simulink model "apertura_chiusura_automatica"  (R2023b)
settings: Solver=VariableStepAuto  StartTime=0.0  StopTime=60  RelTol=1e-3
settings Model: Creator=Asus  LastModifiedBy=Asus
settings OptimizationCC: ReuseModelBlockBuffer=off

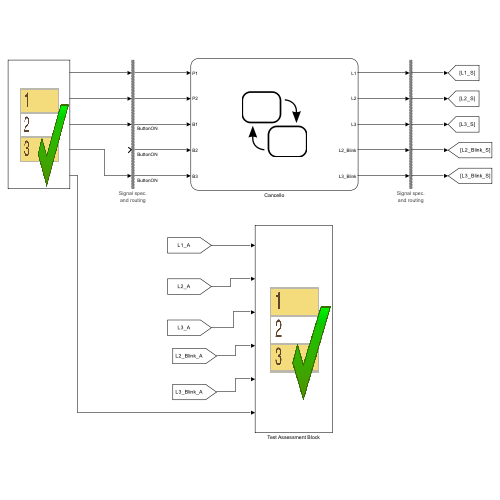
[thumbnail: Simulink's stored preview of the top-level diagram]
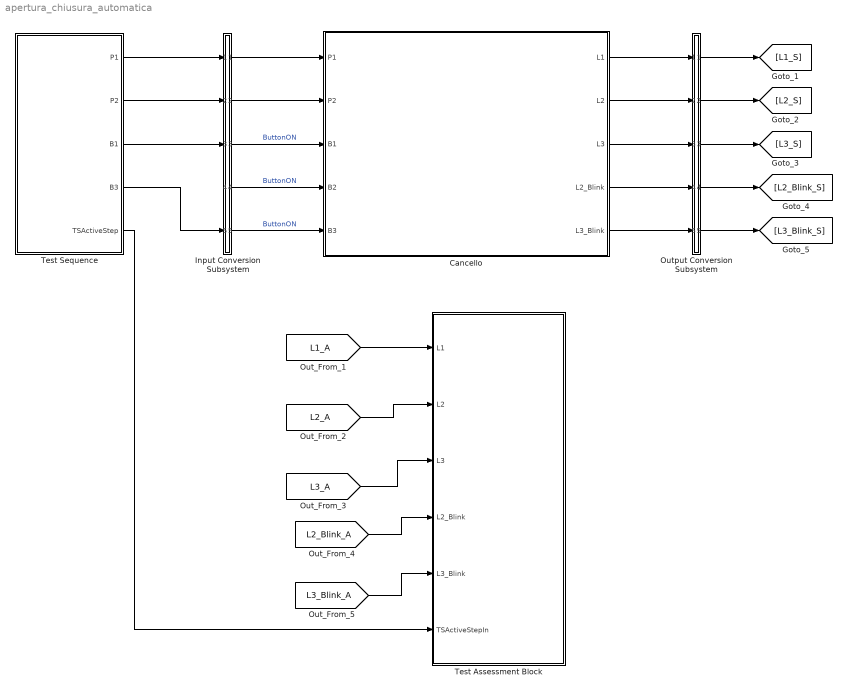
== system apertura_chiusura_automatica ==
  Cancello : Stateflow chart  TreatAsAtomicUnit=on
  Input Conversion Subsystem : Subsystem  Tag=__SLT_ICS__  Description=|
      | Signal spec.
      | and routing
      settings: AttributesFormatString=%<Description>
  Output Conversion Subsystem : Subsystem  Tag=__SLT_OCS__  Description=|
      | Signal spec.
      | and routing
      settings: AttributesFormatString=%<Description>
  Test Assessment Block : Test Sequence  Tag=__SLT_ASMT__  TreatAsAtomicUnit=on
  Test Sequence : Test Sequence  TreatAsAtomicUnit=on
  wires:
  [L1_A] -> Test Assessment Block/1(L1)
  [L2_A] -> Test Assessment Block/2(L2)
  [L3_A] -> Test Assessment Block/3(L3)
  [L2_Blink_A] -> Test Assessment Block/4(L2_Blink)
  [L3_Blink_A] -> Test Assessment Block/5(L3_Blink)
  Test Sequence/1(P1) -> Input Conversion Subsystem/1(Inport_1)
  Test Sequence/2(P2) -> Input Conversion Subsystem/2(Inport_2)
  Test Sequence/3(B1) -> Input Conversion Subsystem/3(Inport_3)
  Output Conversion Subsystem/1(Outport_1) -> [L1_S]
  Output Conversion Subsystem/2(Outport_2) -> [L2_S]
  Output Conversion Subsystem/3(Outport_3) -> [L3_S]
  Output Conversion Subsystem/4(Outport_4) -> [L2_Blink_S]
  Output Conversion Subsystem/5(Outport_5) -> [L3_Blink_S]
  Input Conversion Subsystem/1(Outport_1) -> Cancello/1(P1)
  Input Conversion Subsystem/2(Outport_2) -> Cancello/2(P2)
  Input Conversion Subsystem/3(Outport_3) -> Cancello/3(B1)  "ButtonON"
  Input Conversion Subsystem/4(Outport_4) -> Cancello/4(B2)  "ButtonON"
  Input Conversion Subsystem/5(Outport_5) -> Cancello/5(B3)  "ButtonON"
  Cancello/1(L1) -> Output Conversion Subsystem/1(Inport_1)
  Cancello/2(L2) -> Output Conversion Subsystem/2(Inport_2)
  Cancello/3(L3) -> Output Conversion Subsystem/3(Inport_3)
  Cancello/4(L2_Blink) -> Output Conversion Subsystem/4(Inport_4)
  Cancello/5(L3_Blink) -> Output Conversion Subsystem/5(Inport_5)
  Test Sequence/5(TSActiveStep) -> Test Assessment Block/6(TSActiveStepIn)
  Test Sequence/4(B3) -> Input Conversion Subsystem/5(Inport_5)

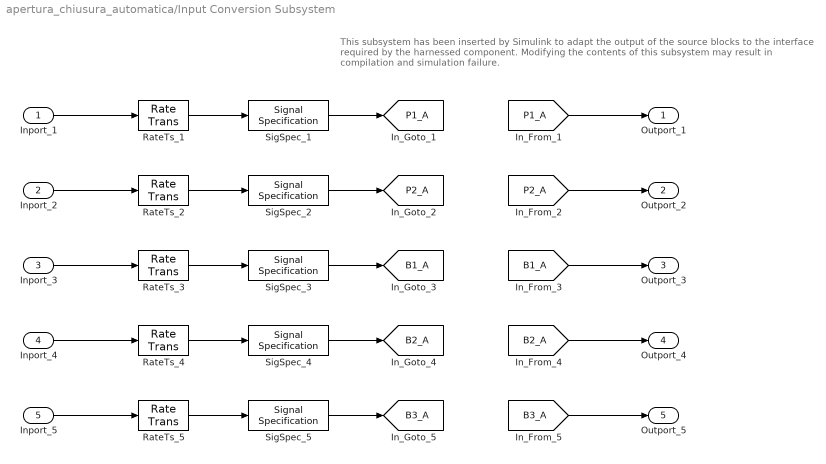
== system apertura_chiusura_automatica/Input Conversion Subsystem ==
  note: This subsystem has been inserted by Simulink to adapt the output of the source blocks to the interface required by the harnessed component.
      |  Modifying the contents of this subsystem may result in compilation and simulation failure.
  Inport_1 : Inport
  Inport_2 : Inport  Port=2
  Inport_3 : Inport  Port=3
  Inport_4 : Inport  Port=4
  Inport_5 : Inport  Port=5
  RateTs_{1..5} (5 alike) : RateTransition  OutPortSampleTime=[0, 1]
  SigSpec_{1..5} (5 alike) : SignalSpecification  OutDataTypeStr=boolean  Dimensions=[1]  SampleTime=[0, 1]
  Outport_1 : Outport
  Outport_2 : Outport  Port=2
  Outport_3 : Outport  Port=3
  Outport_4 : Outport  Port=4
  Outport_5 : Outport  Port=5
  tag scope: B1_A=global, B2_A=global, B3_A=global, P1_A=global, P2_A=global
  wires:
  [P1_A] -> Outport_1/1
  SigSpec_1/1 -> [P1_A]
  RateTs_1/1 -> SigSpec_1/1
  Inport_1/1 -> RateTs_1/1
  [P2_A] -> Outport_2/1
  SigSpec_2/1 -> [P2_A]
  RateTs_2/1 -> SigSpec_2/1
  Inport_2/1 -> RateTs_2/1
  [B1_A] -> Outport_3/1
  SigSpec_3/1 -> [B1_A]
  RateTs_3/1 -> SigSpec_3/1
  Inport_3/1 -> RateTs_3/1
  [B2_A] -> Outport_4/1
  SigSpec_4/1 -> [B2_A]
  RateTs_4/1 -> SigSpec_4/1
  Inport_4/1 -> RateTs_4/1
  [B3_A] -> Outport_5/1
  SigSpec_5/1 -> [B3_A]
  RateTs_5/1 -> SigSpec_5/1
  Inport_5/1 -> RateTs_5/1

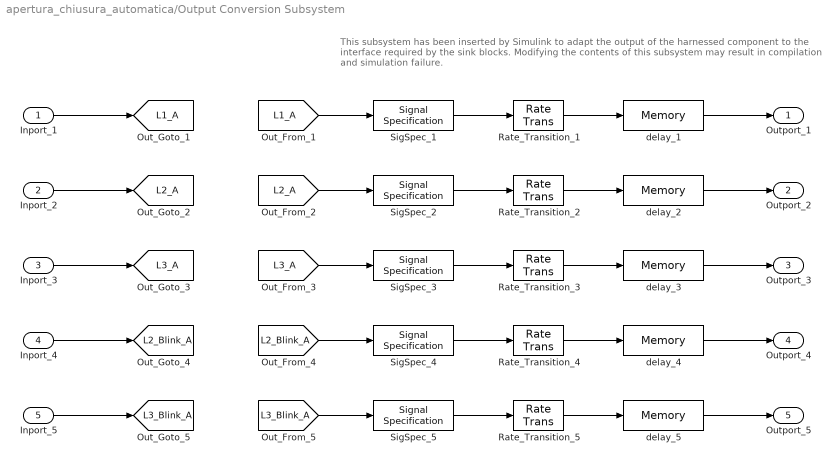
== system apertura_chiusura_automatica/Output Conversion Subsystem ==
  note: This subsystem has been inserted by Simulink to adapt the output of the harnessed component to the interface required by the sink blocks.
      |  Modifying the contents of this subsystem may result in compilation and simulation failure.
  Inport_1 : Inport
  Inport_2 : Inport  Port=2
  Inport_3 : Inport  Port=3
  Inport_4 : Inport  Port=4
  Inport_5 : Inport  Port=5
  Rate_Transition_{1..5} (5 alike) : RateTransition  OutPortSampleTimeOpt=Inherit
  SigSpec_{1..5} (5 alike) : SignalSpecification  OutDataTypeStr=boolean  Dimensions=[1]
  delay_{1..5} (5 alike) : Memory
  Outport_1 : Outport
  Outport_2 : Outport  Port=2
  Outport_3 : Outport  Port=3
  Outport_4 : Outport  Port=4
  Outport_5 : Outport  Port=5
  tag scope: L1_A=global, L2_A=global, L2_Blink_A=global, L3_A=global, L3_Blink_A=global
  wires:
  Inport_1/1 -> [L1_A]
  [L1_A] -> SigSpec_1/1
  SigSpec_1/1 -> Rate_Transition_1/1
  Rate_Transition_1/1 -> delay_1/1
  delay_1/1 -> Outport_1/1
  Inport_2/1 -> [L2_A]
  [L2_A] -> SigSpec_2/1
  SigSpec_2/1 -> Rate_Transition_2/1
  Rate_Transition_2/1 -> delay_2/1
  delay_2/1 -> Outport_2/1
  Inport_3/1 -> [L3_A]
  [L3_A] -> SigSpec_3/1
  SigSpec_3/1 -> Rate_Transition_3/1
  Rate_Transition_3/1 -> delay_3/1
  delay_3/1 -> Outport_3/1
  Inport_4/1 -> [L2_Blink_A]
  [L2_Blink_A] -> SigSpec_4/1
  SigSpec_4/1 -> Rate_Transition_4/1
  Rate_Transition_4/1 -> delay_4/1
  delay_4/1 -> Outport_4/1
  Inport_5/1 -> [L3_Blink_A]
  [L3_Blink_A] -> SigSpec_5/1
  SigSpec_5/1 -> Rate_Transition_5/1
  Rate_Transition_5/1 -> delay_5/1
  delay_5/1 -> Outport_5/1

== stateflow chart apertura_chiusura_automatica/Test Assessment Block ==
  state Run
    state VerifyInit
      verify(~L1 & ~L2 & ~L3 & ~L2_Blink & ~L3_Blink)
    state VerifyIAumentoTimerChiusura
      verify(~L1 & ~L2 & ~L3 & ~L2_Blink & ~L3_Blink)
    state VerifyRichiestaApertura
      verify(~L1 & ~L2 & ~L3 & L2_Blink & ~L3_Blink)
    state VerifyApertura
      verify(~L1 & ~L2 & ~L3 & L2_Blink & ~L3_Blink)
    state VerifyCancelloAperto
      verify(L1 & L2 & L3 & ~L2_Blink & ~L3_Blink)
    state VerifyAvvioTimer
      verify(L1 & L2 & L3 & ~L2_Blink & ~L3_Blink)
    state VerifyAvvioChiusura
      verify(~L1 && ~L2 && ~L3 && L2_Blink && ~L3_Blink)
    state VerifyChiusura
      verify(~L1 && ~L2 && ~L3 && L2_Blink && ~L3_Blink)
    state VerifyCancelloChiuso
      verify(~L1 && ~L2 && ~L3 && ~L2_Blink && ~L3_Blink)
    state Run_1
    (default) -> (junction 22)
    Run -> (junction 22)
    (junction 22) -> (junction 23) [order 1] : [TSActiveStepIn==TSActiveStepEnumH1.Init
        | ]
    (junction 23) -> VerifyInit [order 1] : [~in(Run.VerifyInit)]
    (junction 225) -> (junction 116) [order 2]
    (junction 23) -> (junction 26) [order 2]
    (junction 225) -> (junction 226) [order 1] : [TSActiveStepIn==TSActiveStepEnumH1.AumentoTimerChiusura
        | ]
    (junction 226) -> VerifyIAumentoTimerChiusura [order 1] : [~in(Run.VerifyIAumentoTimerChiusura)]
    (junction 116) -> (junction 117) [order 1] : [TSActiveStepIn==TSActiveStepEnumH1.RichiestaApertura
        | ]
    (junction 117) -> VerifyRichiestaApertura [order 1] : [~in(Run.VerifyRichiestaApertura)]
    (junction 116) -> (junction 146) [order 2]
    (junction 117) -> (junction 120) [order 2]
    (junction 146) -> (junction 147) [order 1] : [TSActiveStepIn==TSActiveStepEnumH1.Apertura
        | ]
    (junction 147) -> VerifyApertura [order 1] : [~in(Run.VerifyApertura)]
    (junction 146) -> (junction 61) [order 2]
    (junction 147) -> (junction 150) [order 2]
    (junction 61) -> (junction 62) [order 1] : [TSActiveStepIn==TSActiveStepEnumH1.CancelloAperto
        | ]
    (junction 62) -> VerifyCancelloAperto [order 1] : [~in(Run.VerifyCancelloAperto)]
    (junction 61) -> (junction 216) [order 2]
    (junction 62) -> (junction 65) [order 2]
    (junction 216) -> (junction 217) [order 1] : [TSActiveStepIn==TSActiveStepEnumH1.AvvioTimer
        | ]
    (junction 217) -> VerifyAvvioTimer [order 1] : [~in(Run.VerifyAvvioTimer)]
    (junction 216) -> (junction 207) [order 2]
    (junction 217) -> (junction 220) [order 2]
    (junction 207) -> (junction 208) [order 1] : [TSActiveStepIn==TSActiveStepEnumH1.AvvioChiusura
        | ]
    (junction 208) -> VerifyAvvioChiusura [order 1] : [~in(Run.VerifyAvvioChiusura)]
    (junction 207) -> (junction 197) [order 2]
    (junction 208) -> (junction 211) [order 2]
    (junction 197) -> (junction 198) [order 1] : [TSActiveStepIn==TSActiveStepEnumH1.Chiusura
        | ]
    (junction 198) -> VerifyChiusura [order 1] : [~in(Run.VerifyChiusura)]
    (junction 197) -> (junction 69) [order 2]
    (junction 198) -> (junction 201) [order 2]
    (junction 69) -> (junction 70) [order 1] : [TSActiveStepIn==TSActiveStepEnumH1.CancelloChiuso
        | ]
    (junction 70) -> VerifyCancelloChiuso [order 1] : [~in(Run.VerifyCancelloChiuso)]
    (junction 69) -> (junction 78) [order 2]
    (junction 70) -> (junction 73) [order 2]
    (junction 78) -> (junction 79)
    (junction 79) -> Run_1 [order 1] : [~in(Run.Run_1)]
    (junction 79) -> (junction 82) [order 2]
    (junction 226) -> (junction 229) [order 2]
    (junction 22) -> (junction 225) [order 2]
  (default) -> Run
  data: L1 input boolean size=[1]; L2 input boolean size=[1]; L3 input boolean size=[1]; L2_Blink input boolean size=[1]; L3_Blink input boolean size=[1]; TSActiveStepIn input

== stateflow chart apertura_chiusura_automatica/Test Sequence ==
  settings: sampleTime=2.4
  state Init
    %% Initialize data outputs.
    P2 = true;
    P1 = false;
    settings: description=Allo step Init il cancello si trova nello Stato di Check dove abbiamo il cancello chiuso e tutti i led spenti.
  state AumentoTimerChiusura
    B3=true;
    settings: description=|
        | A cancello chiuso viene incrementato di dieci secondi il tempo di attesa per la chiusura automatica.
        |  -> in cancello Aperto after(20,sec)
        | non viene testato l'incremento completo da 10 a 120, fino a tornare a 10 secondi
        | in quanto uguale al test apertura_chiusura_automatica
  state RichiestaApertura
    P2 = true;
    B1 = true;
    B3=false;
    settings: description=Con la pressione e il rilascio di B1 richiediamo l'apertura del cancello. il led giallo si attiva
  state Apertura
    B1 =false;
    P2 =false;
    settings: description=|
        | Step che indica il movimento del cancello. il led giallo lampeggia.
        | Questo step ha una durata di  10 secondi (tempo di apertura del cancello di default)
  state CancelloAperto
    B1 =false;
    P2 =false;
    settings: description=Non viene richiesta la di chiusura del cancello tramite B1, quindi il cancello si richiuderà dopo 20 secondi
  state AvvioTimer
    P2 =false;
    settings: description=Avvio del Timer
  state AvvioChiusura
    P2 =false;
    settings: description=Timer scaduto e inizio chiusura automatica
  state Chiusura
    B1 = false;
    settings: description=|
        | Step che indica il movimento del cancello. il led giallo lampeggia.
        | Questo step ha una durata di  10 secondi (tempo di apertura del cancello di default).
        | Nel test apertura_chiusura.automatica verrà illustrata la chiusura automatica
  state CancelloChiuso
    P2 = true;
    B1 = false;
    settings: description=Abbiamo il cancello chiuso e tutti i led spenti
  (default) -> Init
  Init -> AumentoTimerChiusura : [
      | true
      | ]
  AumentoTimerChiusura -> RichiestaApertura : [
      | true
      | ]
  RichiestaApertura -> Apertura : [
      | true
      | ]
  Apertura -> CancelloAperto : [
      | after(10,sec)
      | ]
  CancelloAperto -> AvvioTimer : [
      | after(20,sec)
      | ]
  AvvioTimer -> AvvioChiusura : [
      | true
      | ]
  AvvioChiusura -> Chiusura : [
      | true
      | ]
  Chiusura -> CancelloChiuso : [
      | after(10,sec)
      | ]
  data: P1 output boolean size=[1]; P2 output boolean size=[1]; B1 output boolean size=[1]; B3 output; TSActiveStep output Enum: TSActiveStepEnumH1

== stateflow chart apertura_chiusura_automatica/Cancello ==
  settings: executeAtInitialization=1
  state Cancello [parallel]
    settings: executionOrder=1
    state Check
      en: L1=OFF; L2=OFF; L3=OFF;L2_Blink=OFF;L3_Blink=OFF
    state Error
      state Wait1
      state ERR
        en: L1=ON
        ex: L1=OFF
      (default) -> Wait1
      Wait1 -> ERR : [after(10,sec)]
    state Close
      state Closing
        en:L2_Blink=ON; Start_T_L_C=ON;
        ex:Start_T_L_C=OFF; L2_Blink=OFF;
      state Closed
      (default) -> Closing
      Closing -> Closed : [T_L==ON && P2 == true]
    state Open
      state Opening
        en: Start_T_L_O=ON;L2_Blink=ON;
        ex:L2_Blink=OFF,Start_T_L_O=OFF
      state Opened
        en:L1=ON; L2=ON; L3=ON; Start_T_C=ON;
        du: Reset();
        ex: L1=OFF; L2=OFF; L3=OFF; Start_T_C=OFF;
      (default) -> Opening
      Opening -> Opened : [T_L == ON]
    (default) -> Check
    Check -> Open [order 2] : [B1 == ON && P1 == false || P1 == true && P2 == false]
    Close -> Error [order 2] : [T_L==ON&&P2==false]
    Check -> Close [order 1] : [P1 == false && P2 == false]
    Close -> Open [order 1] : [B1 == ON && P1 == false || in(Close.Closing) && P1==true]
    Error -> Closed : [P2==true]
    Open -> Close : [(B1 == ON || T_C == true) && P1==false]
  state Timer_T_L_O [parallel]
    settings: executionOrder=7
    state Counting
      state Count1
      state End
        en: T_L = ON
      (default) -> Timer_T_L_O.Counting.Count1
      Timer_T_L_O.Counting.Count1 -> Timer_T_L_O.Counting.End [order 1] : [after(Time_T_L,sec)]
      Timer_T_L_O.Counting.Count1 -> Timer_T_L_O.Counting.Count1 [order 2] : [RESET == ON]
    state off
      en: T_L =OFF
    (default) -> Timer_T_L_O.off
    Timer_T_L_O.off -> Timer_T_L_O.Counting : [Start_T_L_O == ON]
    Timer_T_L_O.Counting -> Timer_T_L_O.off : [Start_T_L_O == OFF]
  state Timer_T_L_C [parallel]
    settings: executionOrder=4
    state Counting
      state Count1
      state End
        en: T_L = ON
      (default) -> Timer_T_L_C.Counting.Count1
      Timer_T_L_C.Counting.Count1 -> Timer_T_L_C.Counting.End [order 1] : [after(Time_T_L,sec)]
      Timer_T_L_C.Counting.Count1 -> Timer_T_L_C.Counting.Count1 [order 2] : [RESET == ON]
    state off
      en: T_L =OFF
    (default) -> Timer_T_L_C.off
    Timer_T_L_C.off -> Timer_T_L_C.Counting : [Start_T_L_C == ON]
    Timer_T_L_C.Counting -> Timer_T_L_C.off : [Start_T_L_C == OFF]
  state Reset [function]
    (default) -> (junction 65)
    (junction 65) -> (junction 68) [order 1] : [P1==true]
    (junction 68) -> (junction 73) : {RESET=true;}
    (junction 65) -> (junction 71) [order 2] : [P1==false]
    (junction 71) -> (junction 73) : {RESET=false;}
  state Update_Time_T_L [function]
    (default) -> (junction 97)
    (junction 97) -> (junction 99) [order 1] : [Time_T_L < 120]
    (junction 99) -> (junction 107) : {Time_T_L=Time_T_L+10}
    (junction 97) -> (junction 103) [order 2] : [Time_T_L >= 120]
    (junction 103) -> (junction 107) : {Time_T_L = 10}
  state Timet_T_C [parallel]
    settings: executionOrder=5
    state Counting
      state Count1
      state End
        en: T_C = ON
      (default) -> Timet_T_C.Counting.Count1
      Timet_T_C.Counting.Count1 -> Timet_T_C.Counting.End [order 1] : [after(Time_T_C,sec)]
      Timet_T_C.Counting.Count1 -> Timet_T_C.Counting.Count1 [order 2] : [RESET == ON]
    state off
      en: T_C =OFF
    (default) -> Timet_T_C.off
    Timet_T_C.off -> Timet_T_C.Counting : [Start_T_C == ON]
    Timet_T_C.Counting -> Timet_T_C.off : [Start_T_C == OFF]
  state Update_Time_T_C [function]
    (default) -> (junction 114)
    (junction 114) -> (junction 116) [order 1] : [Time_T_C < 120]
    (junction 116) -> (junction 120) : {Time_T_C=Time_T_C + 10}
    (junction 114) -> (junction 118) [order 2] : [Time_T_C >= 120]
    (junction 118) -> (junction 120) : {Time_T_C = 10}
  state Obstacle [parallel]
    settings: executionOrder=2
    state Wait
    state OBS
      en: L3_Blink=ON;Start_T_LV=ON
      du: Reset_LV()
      ex:L3_Blink=OFF;Start_T_LV=OFF
    (default) -> Wait
    Wait -> OBS : [(in(Cancello.Close.Closed) || in(Cancello.Open.Opened) || in(Cancello.Check)) && B1==ON &&P1==true]
    OBS -> Wait : [P1==false || T_LV==ON ]
  state Update [parallel]
    settings: executionOrder=3
    state Update_TC [parallel]
      settings: executionOrder=1
      state Update_T_C
      state UP_TC
        en: Update_Time_T_C()
      (default) -> Update_T_C
      UP_TC -> Update_T_C
      Update_T_C -> UP_TC : [(in(Cancello.Close.Closed)||in(Cancello.Check)) && B3 == ON]
    state Update_TL [parallel]
      settings: executionOrder=2
      state Update_T_L
      state UP_TL
        en: Update_Time_T_L()
      (default) -> Update_T_L
      UP_TL -> Update_T_L
      Update_T_L -> UP_TL : [(in(Cancello.Close.Closed) || in(Cancello.Check)) && B2==ON]
  state Timer_LV [parallel]
    settings: executionOrder=6
    state Counting
      state Count1
      state End
        en: T_LV = ON
      (default) -> Timer_LV.Counting.Count1
      Timer_LV.Counting.Count1 -> Timer_LV.Counting.End [order 1] : [after(30,sec)]
      Timer_LV.Counting.Count1 -> Timer_LV.Counting.Count1 [order 2] : [RESET_LV==true]
    state off
      en: T_LV =OFF
    (default) -> Timer_LV.off
    Timer_LV.off -> Timer_LV.Counting : [Start_T_LV == ON]
    Timer_LV.Counting -> Timer_LV.off : [Start_T_LV == OFF]
  state Reset_LV [function]
    (default) -> (junction 81)
    (junction 81) -> (junction 83) [order 1] : [B1==ON]
    (junction 81) -> (junction 89) [order 2] : [B1==OFF]
    (junction 83) -> (junction 87) : {RESET_LV=true}
    (junction 89) -> (junction 87) : {RESET_LV=false}
  data: L1 output boolean; L2 output boolean; L3 output boolean; OFF constant boolean =false; P1 input boolean; P2 input boolean; ON constant boolean =true; B1 input boolean; Time_T_C local double =10; Time_T_L local double =10; L2_Blink output boolean; L3_Blink output boolean; B2 input boolean; B3 input boolean; RESET local boolean; Start_T_C local boolean; Start_T_L_O local boolean; T_L local boolean; T_C local boolean; T_LV local boolean; RESET_LV local boolean; Start_T_LV local boolean; Start_T_L_C local double
